simulink model "playback_4khz"  (R2016b)
settings: Solver=FixedStepDiscrete  StartTime=58  StopTime=73  FixedStep=elmo_sample_time  RelTol=1e-3
undefined symbols (not defined in the file or in its folder): elmo_sample_time, sample_time, time_1000_recorded, time_4000_recorded
libraries: simulink x2
settings Model: Creator=wmartin  LastModifiedBy=Will
settings SolverCC: EnableConcurrentExecution=on
settings DataIOCC: MaxDataPoints=1000000000  SaveFormat=StructureWithTime  SignalLogging=off  DSMLogging=off  VisualizeSimOutput=off
settings OptimizationCC: BlockReduction=off  OptimizeBlockIOStorage=off  BufferReuse=off  GlobalBufferReuse=off  ExpressionFolding=off  ExpressionDepthLimit=2147483647  LocalBlockOutputs=off  LifeSpan=inf  SimCompilerOptimization=on
settings DebuggingCC: UnderspecifiedInitializationDetection=Classic  MergeDetectMultiDrivingBlocksExec=none  SolverPrmCheckMsg=warning  StateNameClashWarn=warning  SFUnexpectedBacktrackingDiag=warning  SFNoUnconditionalDefaultTransitionDiag=warning  SFExecutionAtInitializationDiag=none
settings HardwareCC: ProdBitPerPointer=32  ProdBitPerSizeT=32  ProdBitPerPtrDiffT=32  ProdLargestAtomicFloat=None  ProdWordSize=32  ProdLongLongMode=on  ProdHWDeviceType=Generic->32-bit x86 compatible
settings ModelReferenceCC: UpdateModelReferenceTargets=IfOutOfDate  ModelReferenceNumInstancesAllowed=Single  ModelReferenceMinAlgLoopOccurrences=on  PropagateSignalLabelsOutOfModel=off
settings RTWCC: SystemTargetFile=slrt.tlc  TemplateMakefile=slrt_default_tmf  Description=Simulink Real-Time  RTWVerbose=off  RTWCompilerOptimization=on
settings CodeAppCC: MaxIdLength=256
settings SimulinkRealTimeCC: GeneratePreprocessorConditionals=Disable all
settings ConfigComp: CovMetricSettings=dw  CovHtmlReporting=on  CovSaveCumulativeToWorkspaceVar=on  CovSaveSingleToWorkspaceVar=on  CovExternalEMLEnable=off  CovSFcnEnable=off

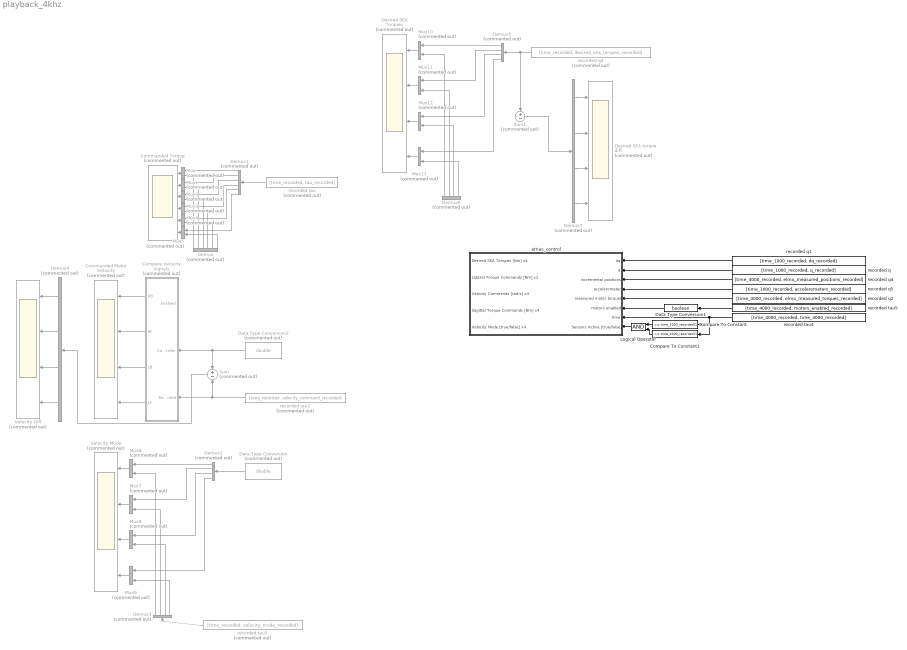
== system playback_4khz ==
  Commanded Motor Velocity : Scope  Commented=on  NumInputPorts=4
  Commanded Torque : Scope  Commented=on  NumInputPorts=6
  Compare To Constant : simulink/Logic and Bit Operations/Compare To Constant  relop=>=  const=time_1000_recorded(1)  OutDataTypeStr=boolean
  Compare To Constant1 : simulink/Logic and Bit Operations/Compare To Constant  relop=>=  const=time_4000_recorded(1)  OutDataTypeStr=boolean
  Compare Velocity Signals : Subsystem  Commented=on
  Data Type Conversion : DataTypeConversion  Commented=on  OutDataTypeStr=double
  Data Type Conversion1 : DataTypeConversion  OutDataTypeStr=boolean
  Data Type Conversion2 : DataTypeConversion  Commented=on  OutDataTypeStr=double
  Demux : Demux  Commented=on  Outputs=6
  Demux1 : Demux  Commented=on  Outputs=6
  Demux{2..7} (6 alike) : Demux  Commented=on
  Desired SEA Torques : Scope  Commented=on  NumInputPorts=4
  Desired SEA torque diff : Scope  Commented=on  NumInputPorts=4
  Logical Operator : Logic  AllPortsSameDT=off  OutDataTypeStr=boolean
  Mux{,1..13} (14 alike) : Mux  Commented=on  Inputs=2
  Sum : Sum  Commented=on  Inputs=+-
  Sum1 : Sum  Commented=on  Inputs=+-
  Velocity Diff : Scope  Commented=on  NumInputPorts=4
  Velocity Mode : Scope  Commented=on  NumInputPorts=4
  atrias_control : Subsystem
  recorded q : FromWorkspace  VariableName=[time_1000_recorded, q_recorded]  OutDataTypeStr=double  SampleTime=sample_time  Interpolate=off  OutputAfterFinalValue=Holding final value
  recorded q1 : FromWorkspace  VariableName=[time_1000_recorded, dq_recorded]  OutDataTypeStr=double  SampleTime=sample_time  Interpolate=off  OutputAfterFinalValue=Holding final value
  recorded q2 : FromWorkspace  VariableName=[time_4000_recorded, elmo_measured_torques_recorded]  OutDataTypeStr=double  SampleTime=elmo_sample_time  Interpolate=off  OutputAfterFinalValue=Holding final value
  recorded q3 : FromWorkspace  Commented=on  VariableName=[time_recorded, desired_sea_torques_recorded]  OutDataTypeStr=double  SampleTime=elmo_sample_time  OutputAfterFinalValue=Holding final value
  recorded q4 : FromWorkspace  VariableName=[time_4000_recorded, elmo_measured_positions_recorded]  OutDataTypeStr=double  SampleTime=elmo_sample_time  Interpolate=off  OutputAfterFinalValue=Holding final value
  recorded q5 : FromWorkspace  VariableName=[time_1000_recorded, accelerometers_recorded]  OutDataTypeStr=double  SampleTime=sample_time  Interpolate=off  OutputAfterFinalValue=Holding final value
  recorded tau : FromWorkspace  Commented=on  VariableName=[time_recorded, tau_recorded]  OutDataTypeStr=double  SampleTime=elmo_sample_time  Interpolate=off  OutputAfterFinalValue=Holding final value
  recorded tau2 : FromWorkspace  Commented=on  VariableName=[time_recorded, velocity_command_recorded]  OutDataTypeStr=double  SampleTime=elmo_sample_time  Interpolate=off  OutputAfterFinalValue=Holding final value
  recorded tau3 : FromWorkspace  Commented=on  VariableName=[time_recorded, velocity_mode_recorded]  OutDataTypeStr=double  SampleTime=elmo_sample_time  Interpolate=off  OutputAfterFinalValue=Holding final value
  recorded tau4 : FromWorkspace  VariableName=[time_4000_recorded, time_4000_recorded]  OutDataTypeStr=double  SampleTime=elmo_sample_time  Interpolate=off  OutputAfterFinalValue=Holding final value
  recorded tau5 : FromWorkspace  VariableName=[time_4000_recorded, motors_enabled_recorded]  OutDataTypeStr=double  SampleTime=elmo_sample_time  Interpolate=off  OutputAfterFinalValue=Holding final value
  wires:
  ? -> Demux/1
  recorded tau/1 -> Demux1/1
  Mux/1 -> Commanded Torque/1
  Mux1/1 -> Commanded Torque/2
  Mux2/1 -> Commanded Torque/3
  Mux3/1 -> Commanded Torque/4
  Mux4/1 -> Commanded Torque/5
  Mux5/1 -> Commanded Torque/6
  Demux1/1 -> Mux/1
  Demux/1 -> Mux/2
  Demux1/2 -> Mux1/1
  Demux1/3 -> Mux2/1
  Demux1/4 -> Mux3/1
  Demux1/5 -> Mux4/1
  Demux1/6 -> Mux5/1
  Demux/2 -> Mux1/2
  Demux/3 -> Mux2/2
  Demux/4 -> Mux3/2
  Demux/5 -> Mux4/2
  Demux/6 -> Mux5/2
  Compare Velocity Signals/1(RB) -> Commanded Motor Velocity/1
  Compare Velocity Signals/2(RF) -> Commanded Motor Velocity/2
  Compare Velocity Signals/3(LB) -> Commanded Motor Velocity/3
  Compare Velocity Signals/4(LF) -> Commanded Motor Velocity/4
  ? -> Compare Velocity Signals/1(Enabled), Data Type Conversion/1
  recorded tau2/1 -> Sum/2, Compare Velocity Signals/3(Recorded)
  Mux6/1 -> Velocity Mode/1
  Mux7/1 -> Velocity Mode/2
  Mux8/1 -> Velocity Mode/3
  Mux9/1 -> Velocity Mode/4
  Demux2/2 -> Mux7/1
  Demux2/3 -> Mux8/1
  Demux2/4 -> Mux9/1
  recorded tau3/1 -> Demux3/1
  Demux3/1 -> Mux6/2
  Demux3/2 -> Mux7/2
  Demux3/3 -> Mux8/2
  Demux3/4 -> Mux9/2
  Data Type Conversion/1 -> Demux2/1
  Demux2/1 -> Mux6/1
  ? -> Data Type Conversion2/1
  Sum/1 -> Demux4/1
  Demux4/4 -> Velocity Diff/4
  Demux4/3 -> Velocity Diff/3
  Demux4/2 -> Velocity Diff/2
  Demux4/1 -> Velocity Diff/1
  Mux10/1 -> Desired SEA Torques/1
  Mux11/1 -> Desired SEA Torques/2
  Mux12/1 -> Desired SEA Torques/3
  Mux13/1 -> Desired SEA Torques/4
  Demux5/2 -> Mux11/1
  Demux5/3 -> Mux12/1
  Demux5/4 -> Mux13/1
  Demux6/1 -> Mux10/2
  Demux6/2 -> Mux11/2
  Demux6/3 -> Mux12/2
  Demux6/4 -> Mux13/2
  recorded q3/1 -> Demux5/1, Sum1/1
  Demux5/1 -> Mux10/1
  ? -> Sum1/2, Demux6/1
  Demux7/3 -> Desired SEA torque diff/3
  Demux7/2 -> Desired SEA torque diff/2
  Demux7/1 -> Desired SEA torque diff/1
  Demux7/4 -> Desired SEA torque diff/4
  Sum1/1 -> Demux7/1
  recorded q/1 -> atrias_control/2(q)
  recorded tau4/1 -> Compare To Constant1/1, Compare To Constant/1, atrias_control/7(time)
  recorded tau5/1 -> Data Type Conversion1/1
  recorded q4/1 -> atrias_control/3(incremental positions)
  Data Type Conversion2/1 -> Sum/1, Compare Velocity Signals/2(Controller)
  Data Type Conversion1/1 -> atrias_control/6(motors enabled)
  recorded q2/1 -> atrias_control/5(measured motor torques)
  recorded q5/1 -> atrias_control/4(accelerometer)
  recorded q1/1 -> atrias_control/1(dq)
  Compare To Constant1/1 -> Logical Operator/2
  Compare To Constant/1 -> Logical Operator/1
  Logical Operator/1 -> atrias_control/8(Sensors Active [true/false])

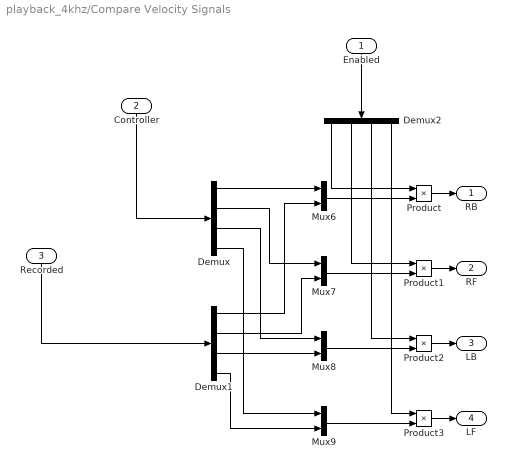
== system playback_4khz/Compare Velocity Signals ==
  Enabled : Inport
  Controller : Inport  Port=2
  Recorded : Inport  Port=3
  Demux : Demux
  Demux1 : Demux
  Demux2 : Demux
  Mux{6..9} (4 alike) : Mux  Inputs=2
  Product{,1..3} (4 alike) : Product
  RB : Outport
  RF : Outport  Port=2
  LB : Outport  Port=3
  LF : Outport  Port=4
  wires:
  Demux/3 -> Mux8/1
  Demux/2 -> Mux7/1
  Demux1/1 -> Mux6/2
  Demux/1 -> Mux6/1
  Product/1 -> RB/1
  Demux/4 -> Mux9/1
  Mux6/1 -> Product/2
  Demux1/4 -> Mux9/2
  Mux7/1 -> Product1/2
  Mux9/1 -> Product3/2
  Recorded/1 -> Demux1/1
  Demux2/3 -> Product2/1
  Demux1/2 -> Mux7/2
  Controller/1 -> Demux/1
  Demux2/1 -> Product/1
  Product3/1 -> LF/1
  Product1/1 -> RF/1
  Product2/1 -> LB/1
  Mux8/1 -> Product2/2
  Demux1/3 -> Mux8/2
  Enabled/1 -> Demux2/1
  Demux2/4 -> Product3/1
  Demux2/2 -> Product1/1

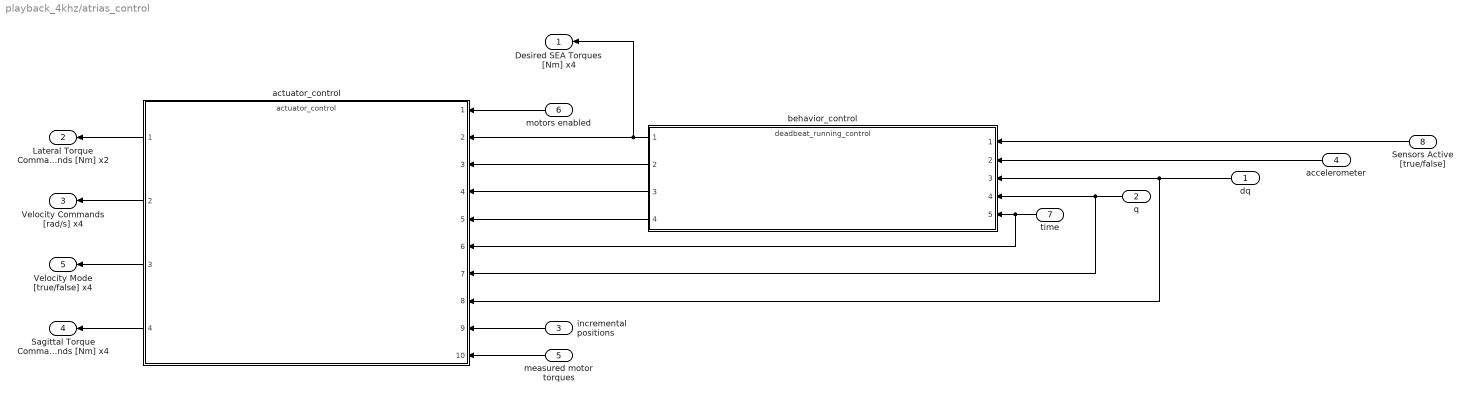
== system playback_4khz/atrias_control ==
  dq : Inport  OutDataTypeStr=double  PortDimensions=13  SampleTime=[0.001,0]
  q : Inport  Port=2  OutDataTypeStr=double  PortDimensions=13  SampleTime=[0.001,0]
  incremental positions : Inport  Port=3  OutDataTypeStr=double  PortDimensions=4  SampleTime=[0.00025000000000000001,0]
  accelerometer : Inport  Port=4  OutDataTypeStr=double  PortDimensions=3  SampleTime=[0.001,0]
  measured motor torques : Inport  Port=5  OutDataTypeStr=double  PortDimensions=4  SampleTime=[0.00025000000000000001,0]
  motors enabled : Inport  Port=6  OutDataTypeStr=boolean  PortDimensions=1  SampleTime=[0.00025000000000000001,0]
  time : Inport  Port=7  OutDataTypeStr=double  PortDimensions=1  SampleTime=[0.00025000000000000001,0]
  Sensors Active [true/false] : Inport  Port=8  PortDimensions=1  SampleTime=[0.001,0]
  actuator_control : ModelReference  ModelNameDialog=actuator_control  SimulationMode=Normal  ModelReferenceVersion=1.1487
  behavior_control : ModelReference  ModelNameDialog=deadbeat_running_control  SimulationMode=Normal  ModelReferenceVersion=1.5050
  Desired SEA Torques [Nm] x4 : Outport  OutDataTypeStr=double  PortDimensions=4  SampleTime=[0.001,0]  InitialOutput=[0 0 0 0]
  Lateral Torque Commands [Nm] x2 : Outport  Port=2  OutDataTypeStr=double  PortDimensions=2  SampleTime=[0.00025000000000000001,0]  InitialOutput=[0 0]
  Velocity Commands [rad/s] x4 : Outport  Port=3  OutDataTypeStr=double  PortDimensions=4  SampleTime=[0.00025000000000000001,0]  InitialOutput=[0 0 0 0]
  Sagittal Torque Commands [Nm] x4 : Outport  Port=4  OutDataTypeStr=double  PortDimensions=4  SampleTime=[0.00025000000000000001,0]  InitialOutput=[0 0 0 0]
  Velocity Mode [true/false] x4 : Outport  Port=5  OutDataTypeStr=boolean  PortDimensions=4  SampleTime=[0.00025000000000000001,0]  InitialOutput=[true true true true]
  wires:
  behavior_control/3 -> actuator_control/4
  behavior_control/4 -> actuator_control/5
  actuator_control/4 -> Sagittal Torque Commands [Nm] x4/1
  actuator_control/2 -> Velocity Commands [rad/s] x4/1
  actuator_control/3 -> Velocity Mode [true/false] x4/1
  Sensors Active [true/false]/1 -> behavior_control/1
  time/1 -> behavior_control/5, actuator_control/6
  q/1 -> behavior_control/4, actuator_control/7
  behavior_control/2 -> actuator_control/3
  behavior_control/1 -> actuator_control/2, Desired SEA Torques [Nm] x4/1
  measured motor torques/1 -> actuator_control/10
  incremental positions/1 -> actuator_control/9
  dq/1 -> behavior_control/3, actuator_control/8
  actuator_control/1 -> Lateral Torque Commands [Nm] x2/1
  accelerometer/1 -> behavior_control/2
  motors enabled/1 -> actuator_control/1
